simulink model "SystemModel"  (R2017b)
settings: Solver=ode45  StartTime=0.0  StopTime=100.0  MaxStep=1  RelTol=1e-3  EnableMultiTasking=on
undefined symbols (not defined in the file): c_p, c_v, epsilon, kappa, lambda_lw, omega_e, p_e, R, T_in, V_d, V_m
settings Model: Creator=baer  LastModifiedBy=niklasbastuck
settings DataIOCC: SaveFormat=Array  SignalLoggingSaveFormat=ModelDataLogs
settings OptimizationCC: ExpressionDepthLimit=2147483647  InitFltsAndDblsToZero=on  LifeSpan=inf
settings DebuggingCC: SaveWithParameterizedLinksMsg=none  UnderspecifiedInitializationDetection=Classic  MergeDetectMultiDrivingBlocksExec=none  SignalResolutionControl=TryResolveAllWithWarning  SolverPrmCheckMsg=warning  MultiTaskDSMMsg=warning  MultiTaskCondExecSysMsg=none  FcnCallInpInsideContextMsg=warning  StateNameClashWarn=warning  SFUnexpectedBacktrackingDiag=warning  SFNoUnconditionalDefaultTransitionDiag=warning  SFExecutionAtInitializationDiag=none
settings HardwareCC: ProdBitPerPointer=32  ProdBitPerSizeT=32  ProdBitPerPtrDiffT=32  ProdLargestAtomicFloat=None  ProdIntDivRoundTo=Undefined  ProdEndianess=Unspecified  ProdWordSize=32  ProdHWDeviceType=32-bit Generic
settings ModelReferenceCC: PropagateSignalLabelsOutOfModel=off
settings CodeAppCC: StateflowObjectComments=on
settings GRTTargetCC: TargetFcnLib=ansi_tfl_tmw.mat  TargetLangStandard=C89/C90 (ANSI)  CombineOutputUpdateFcns=off  GRTInterface=on
settings ConfigComp: CovMetricSettings=dw  CovSaveCumulativeToWorkspaceVar=on  CovSaveSingleToWorkspaceVar=on  CovExternalEMLEnable=off

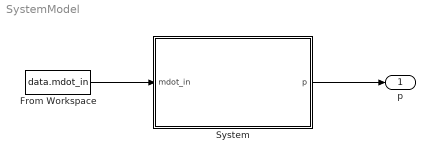
== system SystemModel ==
  From Workspace : FromWorkspace  VariableName=data.mdot_in  ZeroCross=off  OutputAfterFinalValue=Holding final value
  System : Subsystem
  p : Outport  VectorParamsAs1DForOutWhenUnconnected=off
  wires:
  From Workspace/1 -> System/1(mdot_in)
  System/1(p) -> p/1

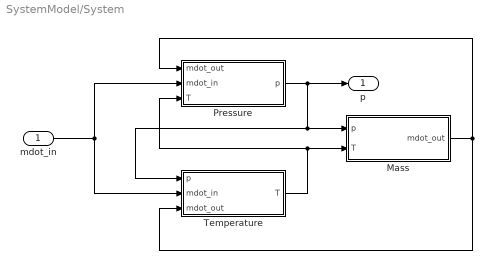
== system SystemModel/System ==
  mdot_in : Inport
  Mass : Subsystem
  Pressure : Subsystem
  Temperature : Subsystem
  p : Outport
  wires:
  Pressure/1(p) -> Temperature/1(p), Mass/1(p), p/1
  Temperature/1(T) -> Mass/2(T), Pressure/3(T)
  Mass/1(mdot_out) -> Temperature/3(mdot_out), Pressure/1(mdot_out)
  mdot_in/1 -> Pressure/2(mdot_in), Temperature/2(mdot_in)

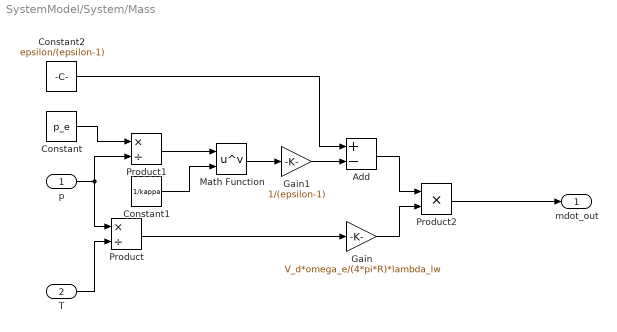
== system SystemModel/System/Mass ==
  p : Inport
  T : Inport  Port=2
  Add : Sum  Inputs=+-
  Constant : Constant  Value=p_e
  Constant1 : Constant  Value=1/kappa
  Constant2 : Constant  Value=epsilon/(epsilon-1)
  Gain : Gain  Gain=V_d*omega_e/(4*pi*R)*lambda_lw
  Gain1 : Gain  Gain=1/(epsilon-1)
  Math Function : Math  Operator=pow  SaturateOnIntegerOverflow=on
  Product : Product  Inputs=*/
  Product1 : Product  Inputs=*/
  Product2 : Product
  mdot_out : Outport
  wires:
  p/1 -> Product/1, Product1/2
  T/1 -> Product/2
  Product/1 -> Gain/1
  Constant/1 -> Product1/1
  Product1/1 -> Math Function/1
  Constant1/1 -> Math Function/2
  Math Function/1 -> Gain1/1
  Gain1/1 -> Add/2
  Constant2/1 -> Add/1
  Add/1 -> Product2/1
  Gain/1 -> Product2/2
  Product2/1 -> mdot_out/1

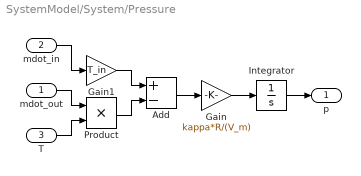
== system SystemModel/System/Pressure ==
  mdot_out : Inport
  mdot_in : Inport  Port=2
  T : Inport  Port=3
  Add : Sum  Inputs=+-
  Gain : Gain  Gain=kappa*R/(V_m)
  Gain1 : Gain  Gain=T_in
  Integrator : Integrator  InitialCondition=30000
  Product : Product
  p : Outport
  wires:
  Add/1 -> Gain/1
  mdot_in/1 -> Gain1/1
  Gain1/1 -> Add/1
  Gain/1 -> Integrator/1
  Integrator/1 -> p/1
  mdot_out/1 -> Product/1
  T/1 -> Product/2
  Product/1 -> Add/2

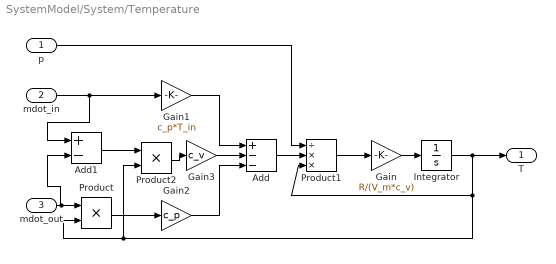
== system SystemModel/System/Temperature ==
  p : Inport
  mdot_in : Inport  Port=2
  mdot_out : Inport  Port=3
  Add : Sum  Inputs=+--
  Add1 : Sum  Inputs=+-
  Gain : Gain  Gain=R/(V_m*c_v)
  Gain1 : Gain  Gain=c_p*T_in
  Gain2 : Gain  Gain=c_p
  Gain3 : Gain  Gain=c_v
  Integrator : Integrator  InitialCondition=300
  Product : Product
  Product1 : Product  Inputs=/**
  Product2 : Product
  T : Outport
  wires:
  mdot_in/1 -> Add1/1, Gain1/1
  Gain1/1 -> Add/1
  mdot_out/1 -> Product/1, Add1/2
  Product/1 -> Gain2/1
  Gain2/1 -> Add/3
  Gain3/1 -> Add/2
  Gain/1 -> Integrator/1
  Integrator/1 -> Product1/3, Product/2, Product2/2, T/1
  Product1/1 -> Gain/1
  Add/1 -> Product1/2
  p/1 -> Product1/1
  Product2/1 -> Gain3/1
  Add1/1 -> Product2/1
